simulink model "a_4"  (R2020a)
settings: Solver=VariableStepAuto  StartTime=0.0  StopTime=1000  RelTol=1e-3
undefined symbols (not defined in the file): A, B, C, Continuous, K_pole, Time, x0
libraries: ctrlSharedLib x1
settings Model: Creator=DEVESH  LastModifiedBy=DEVESH

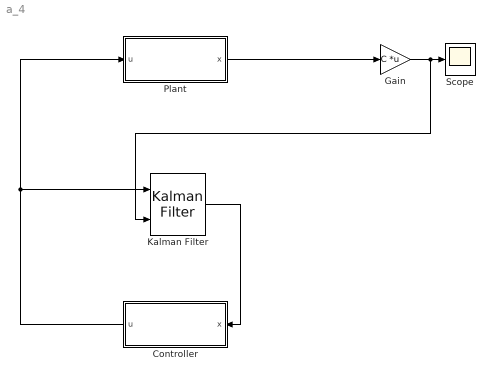
== system a_4 ==
  Controller : Subsystem
  Gain : Gain  Gain=C  Multiplication=Matrix(K*u)
  Kalman Filter : ctrlSharedLib/Kalman Filter  TimeDomain=Continuous-Time  UseCurrentEstimator=on  ModelSource=Individual A, B, C, D matrices  ModelSourceVariable=ss(0.95,1,1,0,1)  A=A  B=B  C=C  D=0  NumberOfStates=1  NumberOfInputs=1  NumberOfOutputs=1  InitialEstimateSource=Dialog  X0=x0  P0=10  UseK=off  UseGH=off  NumberOfProcessNoiseInputs=1  G=1  TimeInvariantG=on  H=0  TimeInvariantH=on  Q=diag([0 0 0 0.005])  TimeInvariantQ=on  R=1  TimeInvariantR=on  N=0  TimeInvariantN=on  AddInputPort=on  AddEnablePort=off  OutputEstimatedY=off  OutputP=off  Ts=-1
  Plant : Subsystem
  Scope : Scope
  wires:
  Plant/1(x) -> Gain/1
  Controller/1(u) -> Plant/1(u), Kalman Filter/1
  Kalman Filter/1 -> Controller/1(x)
  Gain/1 -> Kalman Filter/2, Scope/1

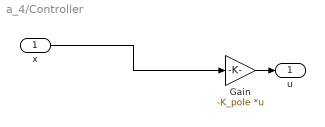
== system a_4/Controller ==
  x : Inport
  Gain : Gain  Gain=-K_pole  Multiplication=Matrix(K*u)
  u : Outport
  wires:
  x/1 -> Gain/1
  Gain/1 -> u/1

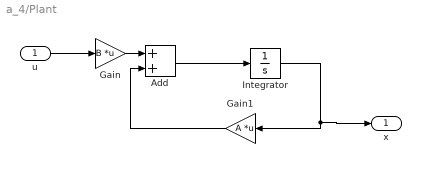
== system a_4/Plant ==
  u : Inport
  Add : Sum
  Gain : Gain  Gain=B  Multiplication=Matrix(K*u)
  Gain1 : Gain  Gain=A  Multiplication=Matrix(K*u)
  Integrator : Integrator  InitialCondition=[0;5*pi/180;0;0]
  x : Outport
  wires:
  u/1 -> Gain/1
  Gain/1 -> Add/1
  Integrator/1 -> x/1, Gain1/1
  Gain1/1 -> Add/2
  Add/1 -> Integrator/1
